simulink model "earthtest"  (Simulink 8.5)
settings: Solver=ode45  SolverMode=SingleTasking  StartTime=0.0  StopTime=1.0  RelTol=1e-3  AbsTol=1e-6
libraries: elements x33
settings Model: Creator=PC  LastModifiedBy=PC  ExtModeTrigMode=oneshot  ExtModeArmWhenConnect=off
settings DataIOCC: LimitDataPoints=off
settings OptimizationCC: BlockReduction=off  BooleanDataType=off  ExpressionDepthLimit=128
settings DebuggingCC: SaveWithParameterizedLinksMsg=none  SignalResolutionControl=TryResolveAllWithWarning  MultiTaskDSMMsg=warning  MultiTaskCondExecSysMsg=none  FcnCallInpInsideContextMsg=EnableAllAsError  StateNameClashWarn=none
settings HardwareCC: TargetUnknown=on

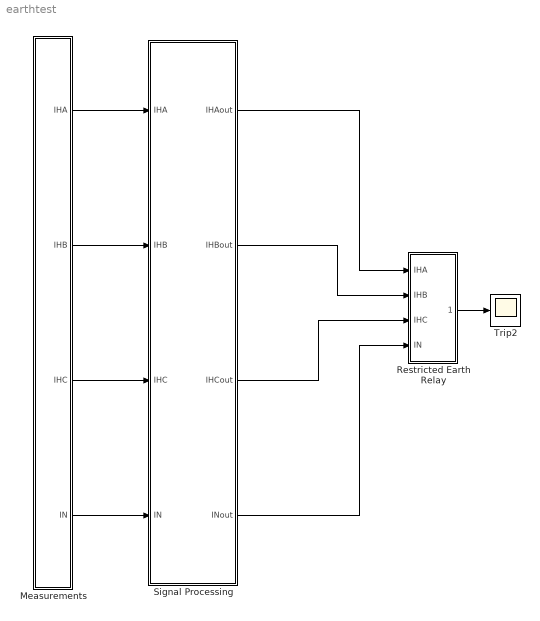
== system earthtest ==
  Measurements : Subsystem
  Restricted Earth Relay : Subsystem  mask(Restricted Earth Protection for the Wye-connected Winding){rc=1, pickup0=0.5, zot=2100, k=0.2, choice=Differential}
      mask prompts: rc "Ratio Mismatch Compensation"; pickup0 "Zero Differential Pick-up Value"; zot "Zero Sequence Overcurrent Threshold"; k "Biased Parameter"; choice "Type of protection"
      mask help: Zero sequence overcurrent protection and zero sequence differential protection.
      mask TypeOptions choice: Overcurrent | Differential
  Signal Processing : Subsystem  mask(Signal Processing){ctx=31.5, cth=1.38, vs=13.8e3, vp=315e3, vector=11}
      mask prompts: ctx "CT Ratio of Low Voltage Side"; cth "CT Ratio of High Voltage Side"; vs "Secondary Voltage"; vp "Primary Voltage"; vector "Transformer Connection Vector"
      mask help: Transform analog measurements to digital format, including filtering, sampling . . .
  Trip2 : Scope
      settings: YMin=-2  YMax=2
  wires:
  Restricted Earth Relay/1(Trip 2) -> Trip2/1
  Measurements/1(IHA) -> Signal Processing/1(IHA)
  Measurements/2(IHB) -> Signal Processing/2(IHB)
  Measurements/3(IHC) -> Signal Processing/3(IHC)
  Measurements/4(IN) -> Signal Processing/4(IN)
  Signal Processing/1(IHAout) -> Restricted Earth Relay/1(IHA)
  Signal Processing/2(IHBout) -> Restricted Earth Relay/2(IHB)
  Signal Processing/3(IHCout) -> Restricted Earth Relay/3(IHC)
  Signal Processing/4(INout) -> Restricted Earth Relay/4(IN)

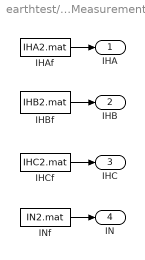
== system earthtest/Measurements ==
  IHAf : FromFile  FileName=IHA2.mat  SampleTime=0
  IHBf : FromFile  FileName=IHB2.mat  SampleTime=0
  IHCf : FromFile  FileName=IHC2.mat  SampleTime=0
  INf : FromFile  FileName=IN2.mat  SampleTime=0
  IHA : Outport
  IHB : Outport  Port=2
  IHC : Outport  Port=3
  IN : Outport  Port=4
  wires:
  IHAf/1 -> IHA/1
  IHBf/1 -> IHB/1
  IHCf/1 -> IHC/1
  INf/1 -> IN/1

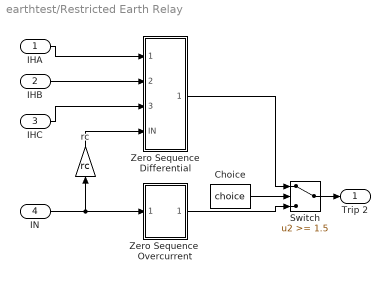
== system earthtest/Restricted Earth Relay ==
  IHA : Inport
  IHB : Inport  Port=2
  IHC : Inport  Port=3
  IN : Inport  Port=4
  Choice : Constant  Value=choice
  Switch : Switch  Threshold=1.5  SaturateOnIntegerOverflow=on  InputSameDT=on
  Zero Sequence Differential : Subsystem
  Zero Sequence  Overcurrent : Subsystem
  rc : Gain  Gain=rc  SaturateOnIntegerOverflow=on  OutDataTypeStr=Inherit: Same as input  ParamDataTypeStr=Inherit: Same as input
  Trip 2 : Outport
  wires:
  Choice/1 -> Switch/2
  Zero Sequence Differential/1(Out1) -> Switch/1
  Switch/1 -> Trip 2/1
  Zero Sequence  Overcurrent/1(Out1) -> Switch/3
  IHA/1 -> Zero Sequence Differential/1(IHA)
  IHB/1 -> Zero Sequence Differential/2(IHB)
  IHC/1 -> Zero Sequence Differential/3(IHC)
  IN/1 -> Zero Sequence  Overcurrent/1(In1), rc/1
  rc/1 -> Zero Sequence Differential/4(IN)

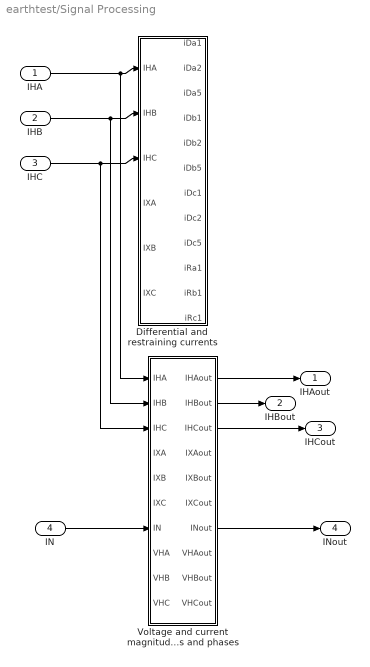
== system earthtest/Signal Processing ==
  IHA : Inport
  IHB : Inport  Port=2
  IHC : Inport  Port=3
  IN : Inport  Port=4
  Differential and  restraining currents : Subsystem
  Voltage and current magnitudes and phases : Subsystem
  IHAout : Outport
  IHBout : Outport  Port=2
  IHCout : Outport  Port=3
  INout : Outport  Port=4
  wires:
  IHA/1 -> Differential and  restraining currents/1(IHA), Voltage and current magnitudes and phases/1(IHA)
  IHB/1 -> Differential and  restraining currents/2(IHB), Voltage and current magnitudes and phases/2(IHB)
  IHC/1 -> Differential and  restraining currents/3(IHC), Voltage and current magnitudes and phases/3(IHC)
  Voltage and current magnitudes and phases/1(IHAout) -> IHAout/1
  Voltage and current magnitudes and phases/2(IHBout) -> IHBout/1
  Voltage and current magnitudes and phases/3(IHCout) -> IHCout/1
  Voltage and current magnitudes and phases/7(INout) -> INout/1
  IN/1 -> Voltage and current magnitudes and phases/7(IN)

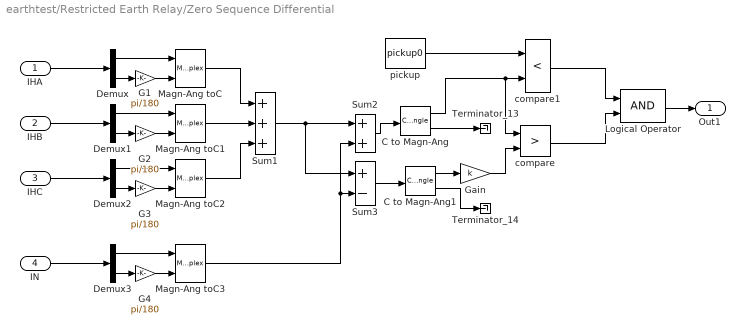
== system earthtest/Restricted Earth Relay/Zero Sequence Differential ==
  IHA : Inport
  IHB : Inport  Port=2
  IHC : Inport  Port=3
  IN : Inport  Port=4
  C to Magn-Ang : ComplexToMagnitudeAngle
  C to Magn-Ang1 : ComplexToMagnitudeAngle
  Demux{,1..3} (4 alike) : Demux  Outputs=2
  G{1..4} (4 alike) : Gain  Gain=pi/180  SaturateOnIntegerOverflow=on  OutDataTypeStr=Inherit: Same as input  ParamDataTypeStr=Inherit: Same as input
  Gain : Gain  Gain=k  SaturateOnIntegerOverflow=on  OutDataTypeStr=Inherit: Same as input  ParamDataTypeStr=Inherit: Same as input
  Logical Operator : Logic
  Magn-Ang toC{,1..3} (4 alike) : MagnitudeAngleToComplex
  Sum1 : Sum  Inputs=+++  SaturateOnIntegerOverflow=on  InputSameDT=on  OutDataTypeStr=Inherit: Same as first input
  Sum2 : Sum  SaturateOnIntegerOverflow=on  InputSameDT=on  OutDataTypeStr=Inherit: Same as first input
  Sum3 : Sum  Inputs=+-  SaturateOnIntegerOverflow=on  InputSameDT=on  OutDataTypeStr=Inherit: Same as first input
  Terminator_13 : Terminator
  Terminator_14 : Terminator
  compare : RelationalOperator  Operator=>  InputSameDT=on
  compare1 : RelationalOperator  Operator=<  InputSameDT=on
  pickup : Constant  Value=pickup0
  Out1 : Outport
  wires:
  Sum2/1 -> C to Magn-Ang/1
  Sum3/1 -> C to Magn-Ang1/1
  IN/1 -> Demux3/1
  Demux3/1 -> Magn-Ang toC3/1
  Magn-Ang toC3/1 -> Sum3/2, Sum2/2
  C to Magn-Ang/2 -> Terminator_13/1
  C to Magn-Ang1/2 -> Terminator_14/1
  C to Magn-Ang1/1 -> Gain/1
  Gain/1 -> compare/2
  Demux3/2 -> G4/1
  G4/1 -> Magn-Ang toC3/2
  pickup/1 -> compare1/1
  C to Magn-Ang/1 -> compare1/2, compare/1
  compare1/1 -> Logical Operator/1
  compare/1 -> Logical Operator/2
  Logical Operator/1 -> Out1/1
  Magn-Ang toC/1 -> Sum1/1
  Sum1/1 -> Sum2/1, Sum3/1
  IHA/1 -> Demux/1
  Demux/1 -> Magn-Ang toC/1
  IHB/1 -> Demux1/1
  Demux1/1 -> Magn-Ang toC1/1
  Magn-Ang toC1/1 -> Sum1/2
  IHC/1 -> Demux2/1
  Demux2/1 -> Magn-Ang toC2/1
  Magn-Ang toC2/1 -> Sum1/3
  Demux/2 -> G1/1
  G1/1 -> Magn-Ang toC/2
  Demux1/2 -> G2/1
  G2/1 -> Magn-Ang toC1/2
  Demux2/2 -> G3/1
  G3/1 -> Magn-Ang toC2/2

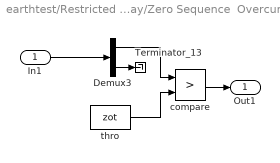
== system earthtest/Restricted Earth Relay/Zero Sequence  Overcurrent ==
  In1 : Inport
  Demux3 : Demux  Outputs=2
  Terminator_13 : Terminator
  compare : RelationalOperator  Operator=>  InputSameDT=on
  thro : Constant  Value=zot
  Out1 : Outport
  wires:
  In1/1 -> Demux3/1
  Demux3/2 -> Terminator_13/1
  thro/1 -> compare/2
  compare/1 -> Out1/1
  Demux3/1 -> compare/1

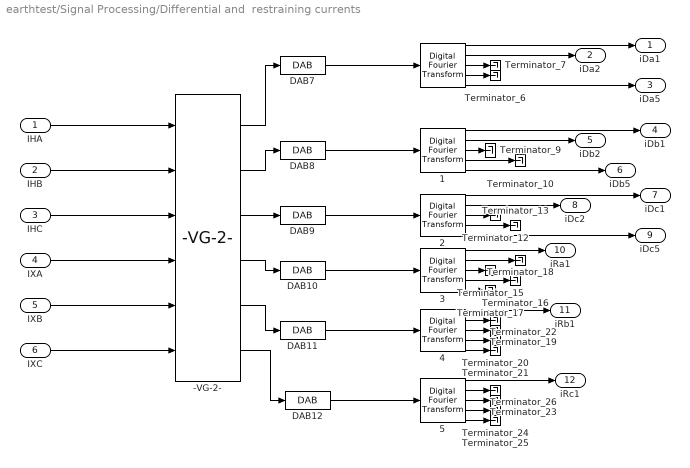
== system earthtest/Signal Processing/Differential and  restraining currents ==
  IHA : Inport
  IHB : Inport  Port=2
  IHC : Inport  Port=3
  IXA : Inport  Port=4
  IXB : Inport  Port=5
  IXC : Inport  Port=6
   {,1..5} (6 alike) : elements/   fo=60  window_size=32  harmonic=[1 2 3 4 5]
  -VG-2- : elements/-VG-2-  trtype=wye - delta  vector=11  Vh=vp  Vx=vs  nCTH=cth  nCTX=ctx
  DAB{8..12} (5 alike) : elements/DAB  filter=off  approx=Bessel  order=2  numerator=[]  denominator=[]  freq=360  resdis=off  vertres=12  xmax=10  winsize=32  G=1.0  fs=60*32
  DAB7 : elements/DAB  filter=on  approx=Bessel  order=2  numerator=[]  denominator=[]  freq=360  resdis=off  vertres=12  xmax=10  winsize=32  G=1.0  fs=60*32
  Terminator_{6..7,9..10,12..13,15..26} (18 alike) : Terminator
  iDa1 : Outport
  iDa2 : Outport  Port=2
  iDa5 : Outport  Port=3
  iDb1 : Outport  Port=4
  iDb2 : Outport  Port=5
  iDb5 : Outport  Port=6
  iDc1 : Outport  Port=7
  iDc2 : Outport  Port=8
  iDc5 : Outport  Port=9
  iRa1 : Outport  Port=10
  iRb1 : Outport  Port=11
  iRc1 : Outport  Port=12
  wires:
  -VG-2-/1 -> DAB7/1
  -VG-2-/2 -> DAB8/1
  -VG-2-/3 -> DAB9/1
  -VG-2-/4 -> DAB10/1
  -VG-2-/5 -> DAB11/1
  -VG-2-/6 -> DAB12/1
  " 2"/3 -> Terminator_12/1
  " 2"/4 -> Terminator_13/1
  " 4"/5 -> Terminator_21/1
  DAB9/1 -> " 2"/1
  " 5"/2 -> Terminator_26/1
  " 5"/3 -> Terminator_23/1
  " 5"/4 -> Terminator_24/1
  " 5"/5 -> Terminator_25/1
  DAB12/1 -> " 5"/1
  " 4"/3 -> Terminator_19/1
  " 4"/2 -> Terminator_22/1
  DAB11/1 -> " 4"/1
  " 4"/4 -> Terminator_20/1
  " 3"/3 -> Terminator_15/1
  " 3"/4 -> Terminator_16/1
  " 3"/5 -> Terminator_17/1
  " 3"/2 -> Terminator_18/1
  DAB10/1 -> " 3"/1
  " 2"/1 -> iDc1/1
  " 2"/2 -> iDc2/1
  " 2"/5 -> iDc5/1
  " 3"/1 -> iRa1/1
  " 4"/1 -> iRb1/1
  " 5"/1 -> iRc1/1
  IXC/1 -> -VG-2-/6
  IXB/1 -> -VG-2-/5
  IXA/1 -> -VG-2-/4
  IHC/1 -> -VG-2-/3
  IHB/1 -> -VG-2-/2
  IHA/1 -> -VG-2-/1
  " "/4 -> Terminator_6/1
  " "/3 -> Terminator_7/1
  DAB7/1 -> " "/1
  " "/1 -> iDa1/1
  " "/2 -> iDa2/1
  " "/5 -> iDa5/1
  " 1"/3 -> Terminator_9/1
  " 1"/4 -> Terminator_10/1
  " 1"/1 -> iDb1/1
  " 1"/2 -> iDb2/1
  " 1"/5 -> iDb5/1
  DAB8/1 -> " 1"/1

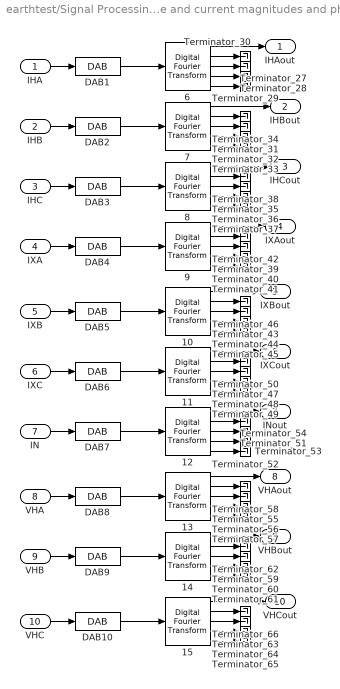
== system earthtest/Signal Processing/Voltage and current magnitudes and phases ==
  IHA : Inport
  IHB : Inport  Port=2
  IHC : Inport  Port=3
  IXA : Inport  Port=4
  IXB : Inport  Port=5
  IXC : Inport  Port=6
  IN : Inport  Port=7
  VHA : Inport  Port=8
  VHB : Inport  Port=9
  VHC : Inport  Port=10
   {6..15} (10 alike) : elements/   fo=60  window_size=32  harmonic=[1 2 3 4 5]
  DAB{1..10} (10 alike) : elements/DAB  filter=off  approx=Bessel  order=2  numerator=[]  denominator=[]  freq=360  resdis=off  vertres=12  xmax=10  winsize=32  G=1.0  fs=60*32
  Terminator_{27..66} (40 alike) : Terminator
  IHAout : Outport
  IHBout : Outport  Port=2
  IHCout : Outport  Port=3
  IXAout : Outport  Port=4
  IXBout : Outport  Port=5
  IXCout : Outport  Port=6
  INout : Outport  Port=7
  VHAout : Outport  Port=8
  VHBout : Outport  Port=9
  VHCout : Outport  Port=10
  wires:
  " 6"/2 -> Terminator_30/1
  " 6"/3 -> Terminator_27/1
  " 6"/4 -> Terminator_28/1
  " 6"/5 -> Terminator_29/1
  DAB1/1 -> " 6"/1
  IHA/1 -> DAB1/1
  " 7"/2 -> Terminator_34/1
  " 7"/3 -> Terminator_31/1
  " 7"/4 -> Terminator_32/1
  " 7"/5 -> Terminator_33/1
  DAB2/1 -> " 7"/1
  " 8"/2 -> Terminator_38/1
  " 8"/3 -> Terminator_35/1
  " 8"/4 -> Terminator_36/1
  " 8"/5 -> Terminator_37/1
  DAB3/1 -> " 8"/1
  " 9"/2 -> Terminator_42/1
  " 9"/3 -> Terminator_39/1
  " 9"/4 -> Terminator_40/1
  " 9"/5 -> Terminator_41/1
  DAB4/1 -> " 9"/1
  " 10"/2 -> Terminator_46/1
  " 10"/3 -> Terminator_43/1
  " 10"/4 -> Terminator_44/1
  " 10"/5 -> Terminator_45/1
  DAB5/1 -> " 10"/1
  " 11"/2 -> Terminator_50/1
  " 11"/3 -> Terminator_47/1
  " 11"/4 -> Terminator_48/1
  " 11"/5 -> Terminator_49/1
  DAB6/1 -> " 11"/1
  " 12"/2 -> Terminator_54/1
  " 12"/3 -> Terminator_51/1
  " 12"/4 -> Terminator_52/1
  " 12"/5 -> Terminator_53/1
  DAB7/1 -> " 12"/1
  " 13"/2 -> Terminator_58/1
  " 13"/3 -> Terminator_55/1
  " 13"/4 -> Terminator_56/1
  " 13"/5 -> Terminator_57/1
  DAB8/1 -> " 13"/1
  " 14"/2 -> Terminator_62/1
  " 14"/3 -> Terminator_59/1
  " 14"/4 -> Terminator_60/1
  " 14"/5 -> Terminator_61/1
  DAB9/1 -> " 14"/1
  " 15"/2 -> Terminator_66/1
  " 15"/3 -> Terminator_63/1
  " 15"/4 -> Terminator_64/1
  " 15"/5 -> Terminator_65/1
  DAB10/1 -> " 15"/1
  " 6"/1 -> IHAout/1
  " 7"/1 -> IHBout/1
  IHB/1 -> DAB2/1
  " 8"/1 -> IHCout/1
  IHC/1 -> DAB3/1
  " 9"/1 -> IXAout/1
  IXA/1 -> DAB4/1
  " 10"/1 -> IXBout/1
  IXB/1 -> DAB5/1
  " 11"/1 -> IXCout/1
  IXC/1 -> DAB6/1
  " 12"/1 -> INout/1
  IN/1 -> DAB7/1
  " 13"/1 -> VHAout/1
  VHA/1 -> DAB8/1
  " 14"/1 -> VHBout/1
  VHB/1 -> DAB9/1
  " 15"/1 -> VHCout/1
  VHC/1 -> DAB10/1
